simulink library "usart_to_cmd"  (R2024b)
settings: Solver=VariableStepAuto  StartTime=0.0  StopTime=10.0  RelTol=1e-3
settings Model: Creator=mainuser  LastModifiedBy=mainuser

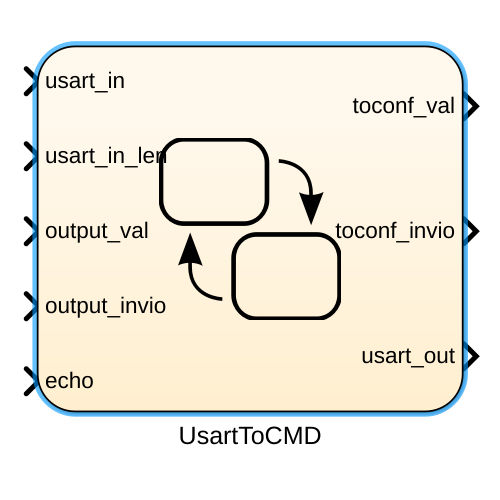
[thumbnail: Simulink's stored preview of the top-level diagram]
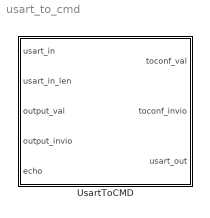
== system usart_to_cmd ==
  UsartToCMD : Stateflow chart  TreatAsAtomicUnit=on

== stateflow chart usart_to_cmd/UsartToCMD ==
  state Wait
  state Send
    en: usart_out=output_val;
    ex: usart_out="";
  state Buffer
    en:
    digited=true;
    value_calc=value_calc*10+(uint64(usart_in)-48);
    if echo
    usart_out=string(char(usart_in));
    end
    ex:
    if echo
    usart_out="";
    end
  state Send1
    en:
    if digited
    toconf_val=uint8(value_calc);
    else
    toconf_val=255;
    end
    digited=false;
    toconf_invio=true;
    if(echo)
    usart_out="" + char(13) + char(10);
    end
    ex:
    toconf_invio=false;
    if(echo)
    usart_out="";
    end
    value_calc=0;
  (default) -> Wait : {value_calc=0;digited=false;}
  (junction 48) -> Wait
  (junction 24) -> Wait [order 2]
  (junction 44) -> (junction 48)
  Wait -> (junction 15)
  Send -> (junction 44)
  (junction 41) -> (junction 44)
  (junction 15) -> Send [order 1] : [output_invio]
  (junction 15) -> (junction 22) [order 2] : [usart_in_len>0]
  (junction 22) -> Buffer [order 1] : [usart_in>=48 && usart_in<=57]
  (junction 22) -> (junction 24) [order 2]
  Buffer -> (junction 41)
  (junction 37) -> (junction 41)
  (junction 24) -> Send1 [order 1] : [usart_in==13]
  Send1 -> (junction 37)
  data: usart_in input uint8 size=1; toconf_val output uint8; toconf_invio output boolean size=1; usart_in_len input uint32 size=1; usart_out output string; output_val input string; output_invio input boolean size=1; echo input boolean size=1; value_calc local uint64 size=1; digited local boolean size=1
